simulink model "prelab2b_block"  (R2018a)
settings: Solver=FixedStepDiscrete  StartTime=0.0  StopTime=20  RelTol=1e-3  EnableMultiTasking=on
values from neighbouring files (symbols this model uses):
  A = 0.1/delta_t    (= 0.2)    [prelab2b.m]    (also in working_data.mat)
  f = 0.9    [prelab2b.m]    (also in working_data.mat)
  kd1 = 1    [prelab2b.m]    (also in working_data.mat)
  kd2 = 1    [prelab2b.m]    (also in working_data.mat)
  kd3 = 1    [prelab2b.m]    (also in working_data.mat)
  kp1 = 150    [prelab2b.m]    (also in working_data.mat)
  kp2 = 150    [prelab2b.m]    (also in working_data.mat)
  kp3 = 150    [prelab2b.m]    (also in working_data.mat)
libraries: legoev3lib x6
settings Model: SimulationMode=external  ExtModeTrigDuration=2  Creator=adityaswaroop  LastModifiedBy=adityaswaroop
settings SolverCC: PositivePriorityOrder=on
settings OptimizationCC: EnhancedBackFolding=on  PassReuseOutputArgsAs=Individual arguments  MaxStackSize=64  OptimizeBlockOrder=speed  DifferentSizesBufferReuse=on  OptimizationCustomize=off
settings DebuggingCC: ParameterTunabilityLossMsg=error
settings HardwareCC: ProdBitPerPointer=32  ProdBitPerSizeT=32  ProdBitPerPtrDiffT=32  ProdLargestAtomicInteger=Long  ProdWordSize=32  ProdHWDeviceType=ARM Compatible->ARM 9
settings SFSimCC: MATLABDynamicMemAlloc=off
settings RTWCC: SystemTargetFile=ert.tlc  HardwareBoard=LEGO MINDSTORMS EV3  TLCOptions="-aInlineSetEventsForThisBaseRateFcn=TLC_FALSE -aSuppressMultiTaskScheduler=TLC_FALSE  -aRateBasedStepFcn=0"  TemplateMakefile=ert_default_tmf  GenerateReport=on  Toolchain=Sourcery G++ Lite v2009q3  IncludeHyperlinkInReport=on  LaunchReport=on  GenerateTraceInfo=on  GenerateTraceReport=on  GenerateTraceReportSl=on  GenerateTraceReportSf=on  GenerateTraceReportEml=on
settings CodeAppCC: ForceParamTrailComments=on  IgnoreCustomStorageClasses=off  OperatorAnnotations=on  SimulinkDataObjDesc=on  SFDataObjDesc=on  InsertBlockDesc=on
settings ERTTargetCC: SupportContinuousTime=on  SupportVariableSizeSignals=on

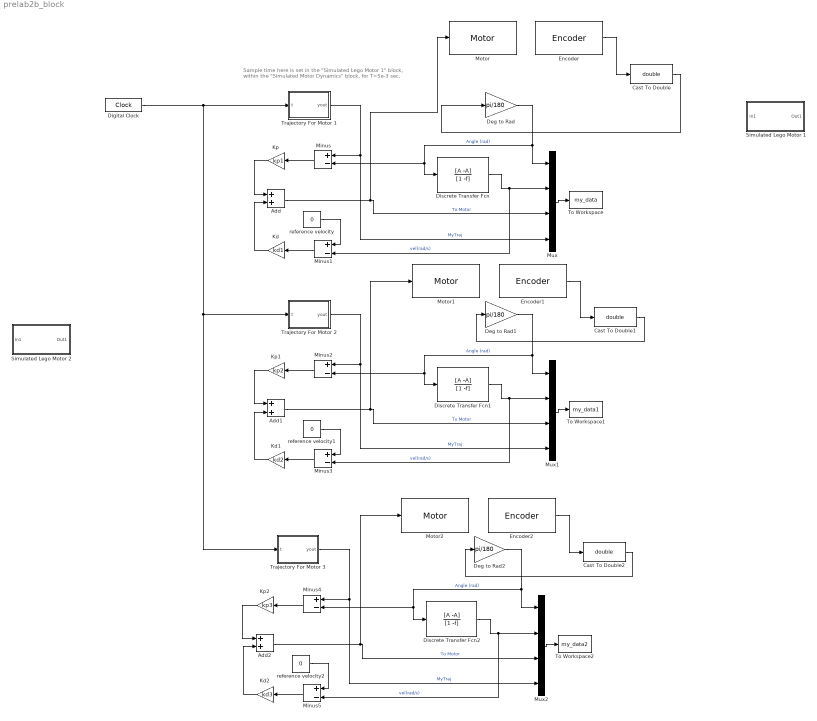
== system prelab2b_block ==
  note: Sample time here is set in the "Simulated Lego Motor 1" block,
      | within the "Simulated Motor Dynamics" block, for T=5e-3 sec.
  Add : Sum
  Add1 : Sum
  Add2 : Sum
  Cast To Double : DataTypeConversion  OutDataTypeStr=double
  Cast To Double1 : DataTypeConversion  OutDataTypeStr=double
  Cast To Double2 : DataTypeConversion  OutDataTypeStr=double
  Deg to Rad : Gain  Gain=pi/180
  Deg to Rad1 : Gain  Gain=pi/180
  Deg to Rad2 : Gain  Gain=pi/180
  Digital Clock : DigitalClock  SampleTime=5e-3
  Discrete Transfer Fcn : DiscreteTransferFcn  Numerator=[A -A]  Denominator=[1 -f]
  Discrete Transfer Fcn1 : DiscreteTransferFcn  Numerator=[A -A]  Denominator=[1 -f]
  Discrete Transfer Fcn2 : DiscreteTransferFcn  Numerator=[A -A]  Denominator=[1 -f]
  Encoder : legoev3lib/Encoder  portNumber=A  opMode=No reset  sampleTime=0.005
      settings: SourceProductName=Simulink Support Package for LEGO MINDSTORMS EV3 Hardware  SourceProductBaseCode=LEGOEV3
  Encoder1 : legoev3lib/Encoder  portNumber=B  opMode=No reset  sampleTime=0.005
      settings: SourceProductName=Simulink Support Package for LEGO MINDSTORMS EV3 Hardware  SourceProductBaseCode=LEGOEV3
  Encoder2 : legoev3lib/Encoder  portNumber=C  opMode=No reset  sampleTime=0.005
      settings: SourceProductName=Simulink Support Package for LEGO MINDSTORMS EV3 Hardware  SourceProductBaseCode=LEGOEV3
  Kd : Gain  Gain=kd1
  Kd1 : Gain  Gain=kd2
  Kd2 : Gain  Gain=kd3
  Kp : Gain  Gain=kp1
  Kp1 : Gain  Gain=kp2
  Kp2 : Gain  Gain=kp3
  Minus{,1..5} (6 alike) : Sum  Inputs=+-
  Motor : legoev3lib/Motor  sportNumber=A  sstopAction=Brake
  Motor1 : legoev3lib/Motor  sportNumber=B  sstopAction=Brake
  Motor2 : legoev3lib/Motor  sportNumber=C  sstopAction=Brake
  Mux : Mux
  Mux1 : Mux
  Mux2 : Mux
  Simulated Lego Motor 1 : Subsystem
  Simulated Lego Motor 2 : Subsystem
  To Workspace : ToWorkspace  VariableName=my_data  SaveFormat=Structure With Time  SampleTime=-1
  To Workspace1 : ToWorkspace  VariableName=my_data1  SaveFormat=Structure With Time  SampleTime=-1
  To Workspace2 : ToWorkspace  VariableName=my_data2  SaveFormat=Structure With Time  SampleTime=-1
  Trajectory For Motor 1 : MATLAB Function  TreatAsAtomicUnit=on
  Trajectory For Motor 2 : MATLAB Function  TreatAsAtomicUnit=on
  Trajectory For Motor 3 : MATLAB Function  TreatAsAtomicUnit=on
  reference velocity : Constant  Value=0
  reference velocity1 : Constant  Value=0
  reference velocity2 : Constant  Value=0
  wires:
  Cast To Double1/1 -> Deg to Rad1/1
  Discrete Transfer Fcn1/1 -> Minus3/2, Mux1/2  "vel(rad/s)"
  Cast To Double/1 -> Deg to Rad/1
  Encoder1/1 -> Cast To Double1/1
  Encoder/1 -> Cast To Double/1
  reference velocity1/1 -> Minus3/1
  Add/1 -> Motor/1, Mux/3  "To Motor"
  Kp1/1 -> Add1/1
  Trajectory For Motor 2/1(yout) -> Mux1/4, Minus2/1  "MyTraj"
  Deg to Rad/1 -> Discrete Transfer Fcn/1, Minus/2, Mux/1  "Angle (rad)"
  reference velocity/1 -> Minus1/1
  Mux1/1 -> To Workspace1/1
  Minus2/1 -> Kp1/1
  Kd1/1 -> Add1/2
  Discrete Transfer Fcn/1 -> Minus1/2, Mux/2  "vel(rad/s)"
  Minus1/1 -> Kd/1
  Kd/1 -> Add/2
  Mux/1 -> To Workspace/1
  Minus/1 -> Kp/1
  Deg to Rad1/1 -> Discrete Transfer Fcn1/1, Minus2/2, Mux1/1  "Angle (rad)"
  Minus3/1 -> Kd1/1
  Trajectory For Motor 1/1(yout) -> Mux/4, Minus/1  "MyTraj"
  Add1/1 -> Motor1/1, Mux1/3  "To Motor"
  Kp/1 -> Add/1
  reference velocity2/1 -> Minus5/1
  Kp2/1 -> Add2/1
  Minus5/1 -> Kd2/1
  Minus4/1 -> Kp2/1
  Add2/1 -> Motor2/1, Mux2/3  "To Motor"
  Deg to Rad2/1 -> Discrete Transfer Fcn2/1, Minus4/2, Mux2/1  "Angle (rad)"
  Digital Clock/1 -> Trajectory For Motor 3/1(t), Trajectory For Motor 2/1(t), Trajectory For Motor 1/1(t)
  Mux2/1 -> To Workspace2/1
  Discrete Transfer Fcn2/1 -> Minus5/2, Mux2/2  "vel(rad/s)"
  Cast To Double2/1 -> Deg to Rad2/1
  Kd2/1 -> Add2/2
  Trajectory For Motor 3/1(yout) -> Mux2/4, Minus4/1  "MyTraj"
  Encoder2/1 -> Cast To Double2/1

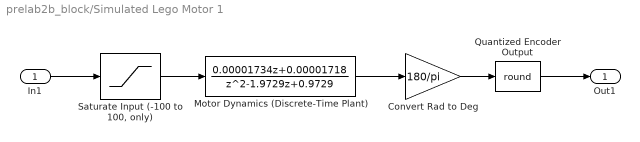
== system prelab2b_block/Simulated Lego Motor 1 ==
  In1 : Inport
  Convert Rad to Deg : Gain  Gain=180/pi
  Motor Dynamics (Discrete-Time Plant) : DiscreteTransferFcn  Numerator="[0.00001734  0.00001718]"  Denominator="[1   -1.9729    0.9729]"
  Quantized Encoder Output : Rounding  Operator=round
  "Saturate Input (-100 to 100, only)" : Saturate  UpperLimit=100  LowerLimit=-100
  Out1 : Outport  VectorParamsAs1DForOutWhenUnconnected=on
  wires:
  In1/1 -> "Saturate Input (-100 to 100, only)"/1
  "Saturate Input (-100 to 100, only)"/1 -> Motor Dynamics (Discrete-Time Plant)/1
  Convert Rad to Deg/1 -> Quantized Encoder Output/1
  Motor Dynamics (Discrete-Time Plant)/1 -> Convert Rad to Deg/1
  Quantized Encoder Output/1 -> Out1/1

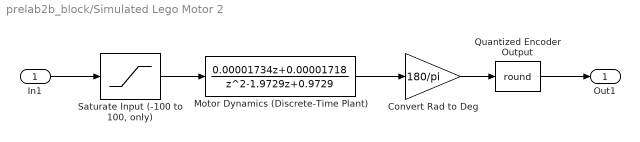
== system prelab2b_block/Simulated Lego Motor 2 ==
  In1 : Inport
  Convert Rad to Deg : Gain  Gain=180/pi
  Motor Dynamics (Discrete-Time Plant) : DiscreteTransferFcn  Numerator="[0.00001734  0.00001718]"  Denominator="[1   -1.9729    0.9729]"
  Quantized Encoder Output : Rounding  Operator=round
  "Saturate Input (-100 to 100, only)" : Saturate  UpperLimit=100  LowerLimit=-100
  Out1 : Outport  VectorParamsAs1DForOutWhenUnconnected=on
  wires:
  In1/1 -> "Saturate Input (-100 to 100, only)"/1
  "Saturate Input (-100 to 100, only)"/1 -> Motor Dynamics (Discrete-Time Plant)/1
  Convert Rad to Deg/1 -> Quantized Encoder Output/1
  Motor Dynamics (Discrete-Time Plant)/1 -> Convert Rad to Deg/1
  Quantized Encoder Output/1 -> Out1/1

== matlab function prelab2b_block/Trajectory For Motor 2 ==
  data: t input; yout output
function yout = MyTrajectory(t)

joint_traj=[0.264668390865136,0.475799229692313,0.632500097122313,0.733915468041950,0.779227079331776,0.767657541793522,0.698477947409933,0.571020384370171,0.384696451761279,0.139023049505138,-0.166343119018979,-0.531560797605545,-0.956547681966371,-1.44091093857329,-1.98386409752323,-2.58413074680076,-3.23983709708612,-3.94839774439829,-4.70640176434860,-5.50950942949176,-6.35237304396499,-7.22859822411347,-8.13076373950116,-9.05051743306729,-9.97876057140313,-10.9059210879712,-11.8222978755043,-12.7184385291808,-13.5855002779176,-14.4155452341083,-15.2017367552290,-15.9384267905132,-16.6211453795314,-17.2465167269894,-17.8121302332924,-18.3163918872352,-18.7583750442921,-19.1376826976688,-19.4543275277520,-19.7086318446274,-19.9011469318351,-20.0325899052172,-20.1037956290301,-20.1156811584521,-20.0692203709455,-19.9654267585711,-19.8053426908289,-19.5900337758489,-19.3205872253348];
ti = linspace(0,20,560);
yi = joint_traj;
yout = interp1(ti,yi,t);
end

== matlab function prelab2b_block/Trajectory For Motor 1 ==
  data: t input; yout output
function yout = MyTrajectory(t)
joint_traj=[-0.652803856585758,-1.30111368649488,-1.94309823046571,-2.57646452432608,-3.19842293907151,-3.80565181137923,-4.39426197690334,-4.95976197848045,-5.49702541498042,-6.00026291146209,-6.46300263220575,-6.87808523449231,-7.23768175491653,-7.53334612075865,-7.75611756485370,-7.89669157787253,-7.94567991241187,-7.89397848246845,-7.73325391505730,-7.45654201650316,-7.05892307881366,-6.53820258277509,-5.89549104770135,-5.13555962148762,-4.26686515213649,-3.30119616431405,-2.25297594450427,-1.13833980991700,0.0258520224875858,1.22291167968450,2.43702518725493,3.65371660273329,4.86008783391250,6.04488000190154,7.19841272077757,8.31245290608113,9.38005282389274,10.3953840361021,11.3535828438205,12.2506147893279,13.0831605667500,13.8485226723437,14.5445506076994,15.1695818677134,15.7223958955512,16.2021784057945,16.6084938057159,16.9412637944238,17.2007505454933];
ti = linspace(0,20,560);
yi = joint_traj;
yout = interp1(ti,yi,t); 
 end

== matlab function prelab2b_block/Trajectory For Motor 3 ==
  data: t input; yout output
function yout = MyTrajectory(t)
joint_traj=[0.264668390865136,0.475799229692313,0.632500097122313,0.733915468041950,0.779227079331776,0.767657541793522,0.698477947409933,0.571020384370171,0.384696451761279,0.139023049505138,-0.166343119018979,-0.531560797605545,-0.956547681966371,-1.44091093857329,-1.98386409752323,-2.58413074680076,-3.23983709708612,-3.94839774439829,-4.70640176434860,-5.50950942949176,-6.35237304396499,-7.22859822411347,-8.13076373950116,-9.05051743306729,-9.97876057140313,-10.9059210879712,-11.8222978755043,-12.7184385291808,-13.5855002779176,-14.4155452341083,-15.2017367552290,-15.9384267905132,-16.6211453795314,-17.2465167269894,-17.8121302332924,-18.3163918872352,-18.7583750442921,-19.1376826976688,-19.4543275277520,-19.7086318446274,-19.9011469318351,-20.0325899052172,-20.1037956290301,-20.1156811584521,-20.0692203709455,-19.9654267585711,-19.8053426908289,-19.5900337758489,-19.3205872253348];
ti = linspace(0,20,560);
yi = joint_traj;
yout = interp1(ti,yi,t);
